simulink model "soft_continuum_model_2_sec"  (R2022a)
settings: Solver=VariableStepAuto  StartTime=0.0  StopTime=4  FixedStep=0.1  RelTol=1e-2
values from neighbouring files (symbols this model uses):
  D = diag([D_1,D_2,D_3,D_4,D_5,D_6])    [workspace_variables.m]
  E_1 = 8.25 * 10^4    (= 82500)    [workspace_variables.m]
  E_2 = 8.25 * 10^4    (= 82500)    [workspace_variables.m]
  g = [g_x,g_y,g_z]    [workspace_variables.m]
  Gs_1 = E_1 / ( 2 * ( 1 + ni) )    (= 27500)    [workspace_variables.m]
  Gs_2 = E_2 / ( 2 *( 1 + ni) )    (= 27500)    [workspace_variables.m]
  Ia_1 = diag([Iax_1,Iay_1,Iaz_1])    [workspace_variables.m]
  Ia_2 = diag([Iax_2,Iay_2,Iaz_2])    [workspace_variables.m]
  Im_1 = diag([Imx_1,Imy_1,Imz_1])    [workspace_variables.m]
  Im_2 = diag([Imx_2,Imy_2,Imz_2])    [workspace_variables.m]
  l_1 = 0.05    [workspace_variables.m]
  l_2 = 0.05    [workspace_variables.m]
  m_1 = 0.08    [workspace_variables.m]
  m_2 = 0.08    [workspace_variables.m]
  q_0 = [0.01 , 0 , 0 , 0.001, 0, 0.0]'    [workspace_variables.m]
  q_dot_0 = [0 , 0, 0, 0, 0, 0]'    [workspace_variables.m]
  t1_p = [0.025  , 0 , 0]    [workspace_variables.m]
  t2_p = [-0.025  , 0 , 0]    [workspace_variables.m]
  t3_p = [0  , 0.025 , 0]    [workspace_variables.m]
  t4_p = [0  , -0.025 , 0]    [workspace_variables.m]
  t5_p = [0.015  , 0 , 0]    [workspace_variables.m]
  twt = pi / 4    (= 0.785398163397)    [workspace_variables.m]
libraries: matrix_library x4, slpidlib x3, dspinverses x3
(part 2 of 2)

== matlab function soft_continuum_model_2_sec/robot model/Subsystem/MATLAB Function1 ==
  data: A input; y output
function y = fcn(A)
 y = cond(A)

== matlab function soft_continuum_model_2_sec/control/PD/Tendons1/Tendons/Subsystem/MATLAB Function1 ==
  data: q input; T_01 output; T_02 output; l_1 input; l_2 input
function [T_01,T_02] = fcn(q,l_1,l_2)
    k_1 = q(1);
    b_1 = q(2);
    t_1 = q(3);
    k_2 = q(4);
    b_2 = q(5);
    t_2 = q(6);
    T1 = T_1(b_1,k_1,l_1,t_1);
    T2 = T_2(b_2,k_2,l_2,t_2);

    T_01 = T1;
    T_02 = T1 * T2;

== matlab function soft_continuum_model_2_sec/Subsystem/Subsystem1/MATLAB Function ==
  data: m_1 input; J1_n output; J2_n output; G_n output; B_n output; C_n output; D_n output; m_2 input; Im_1 input; Im_2 input; l_1 input; l_2 input; Ia_1 input; Ia_2 input; D input; E_1 input; E_2 input; Gs_1 input; Gs_2 input; g input; q input; q_dot input
function [J1_n,J2_n,G_n,B_n,C_n,D_n] = DYNAMIC_MATRICES(m_1,m_2,Im_1,Im_2,l_1,l_2,Ia_1,Ia_2,D,E_1,E_2,Gs_1,Gs_2,g,q,q_dot)

k_1 = q(1);
b_1 = q(2);
t_1 = q(3);
k_2 = q(4);
b_2 = q(5);
t_2 = q(6);

k_dot_1 = q_dot(1);
b_dot_1 = q_dot(2);
t_dot_1 = q_dot(3);
k_dot_2 = q_dot(4);
b_dot_2 = q_dot(5);
t_dot_2 = q_dot(6);

Iax_1 = Ia_1(1,1);
Iay_1 = Ia_1(2,2);
Iaz_1 = Ia_1(3,3);

Iax_2 = Ia_2(1,1);
Iay_2 = Ia_2(2,2);
Iaz_2 = Ia_2(3,3);

Imx_1 = Im_1(1,1);
Imy_1 = Im_1(2,2);
Imz_1 = Im_1(3,3);

Imx_2 = Im_2(1,1);
Imy_2 = Im_2(2,2);
Imz_2 = Im_2(3,3);


g_x = g(1);
g_y = g(2);
g_z = g(3);

C_1_1 = C11(Imx_1,Imx_2,Imy_1,Imy_2,Imz_1,Imz_2,b_1,b_2,b_dot_1,b_dot_2,k_1,k_2,k_dot_1,k_dot_2,l_1,l_2,m_1,m_2,t_1,t_2,t_dot_1,t_dot_2);
C_1_2 = C12(Imx_1,Imx_2,Imy_1,Imy_2,Imz_1,Imz_2,b_1,b_2,b_dot_1,b_dot_2,k_1,k_2,k_dot_1,k_dot_2,l_1,l_2,m_1,m_2,t_1,t_2,t_dot_1,t_dot_2);
C_1_3 = C13(Imx_1,Imx_2,Imy_1,Imy_2,Imz_1,Imz_2,b_1,b_2,b_dot_1,b_dot_2,k_1,k_2,k_dot_1,k_dot_2,l_1,l_2,m_1,m_2,t_1,t_2,t_dot_1,t_dot_2);
C_1_4 = C14(Imx_2,Imy_2,Imz_2,b_1,b_2,b_dot_1,b_dot_2,k_1,k_2,k_dot_1,k_dot_2,l_1,l_2,m_2,t_1,t_2,t_dot_1,t_dot_2);
C_1_5 = C15(Imx_2,Imy_2,Imz_2,b_1,b_2,b_dot_1,b_dot_2,k_1,k_2,k_dot_1,k_dot_2,l_1,l_2,m_2,t_1,t_2,t_dot_1,t_dot_2);
C_1_6 = C16(Imx_2,Imy_2,Imz_2,b_1,b_2,b_dot_1,b_dot_2,k_1,k_2,k_dot_1,k_dot_2,l_1,l_2,m_2,t_1,t_2,t_dot_1,t_dot_2);

C_2_1 = C21(Imx_1,Imx_2,Imy_1,Imy_2,Imz_1,Imz_2,b_1,b_2,b_dot_1,b_dot_2,k_1,k_2,k_dot_1,k_dot_2,l_1,l_2,m_1,m_2,t_1,t_2,t_dot_1,t_dot_2);
C_2_2 = C21(Imx_1,Imx_2,Imy_1,Imy_2,Imz_1,Imz_2,b_1,b_2,b_dot_1,b_dot_2,k_1,k_2,k_dot_1,k_dot_2,l_1,l_2,m_1,m_2,t_1,t_2,t_dot_1,t_dot_2);
C_2_3 = C21(Imx_1,Imx_2,Imy_1,Imy_2,Imz_1,Imz_2,b_1,b_2,b_dot_1,b_dot_2,k_1,k_2,k_dot_1,k_dot_2,l_1,l_2,m_1,m_2,t_1,t_2,t_dot_1,t_dot_2);
C_2_4 = C26(Imx_2,Imy_2,Imz_2,b_1,b_2,b_dot_1,b_dot_2,k_1,k_2,k_dot_1,k_dot_2,l_1,l_2,m_2,t_1,t_2,t_dot_1,t_dot_2);
C_2_5 = C26(Imx_2,Imy_2,Imz_2,b_1,b_2,b_dot_1,b_dot_2,k_1,k_2,k_dot_1,k_dot_2,l_1,l_2,m_2,t_1,t_2,t_dot_1,t_dot_2);
C_2_6 = C26(Imx_2,Imy_2,Imz_2,b_1,b_2,b_dot_1,b_dot_2,k_1,k_2,k_dot_1,k_dot_2,l_1,l_2,m_2,t_1,t_2,t_dot_1,t_dot_2);

C_3_1 = C31(Imx_1,Imx_2,Imy_1,Imy_2,Imz_1,Imz_2,b_1,b_2,b_dot_1,b_dot_2,k_1,k_2,k_dot_1,k_dot_2,l_1,l_2,m_1,m_2,t_1,t_2,t_dot_1,t_dot_2);
C_3_2 = C32(Imx_1,Imx_2,Imy_1,Imy_2,Imz_1,Imz_2,b_1,b_2,b_dot_1,b_dot_2,k_1,k_2,k_dot_1,k_dot_2,l_1,l_2,m_1,m_2,t_1,t_2,t_dot_1,t_dot_2);
C_3_3 = C33(Imx_1,Imx_2,Imy_1,Imy_2,Imz_1,Imz_2,b_1,b_2,b_dot_1,b_dot_2,k_1,k_2,k_dot_1,k_dot_2,l_1,l_2,m_1,m_2,t_1,t_2,t_dot_1,t_dot_2);
C_3_4 =C34(Imx_2,Imy_2,Imz_2,b_1,b_2,b_dot_1,b_dot_2,k_1,k_2,k_dot_1,k_dot_2,l_1,l_2,m_2,t_1,t_2,t_dot_1,t_dot_2);
C_3_5 = C35(Imx_2,Imy_2,Imz_2,b_1,b_2,b_dot_1,b_dot_2,k_1,k_2,k_dot_1,k_dot_2,l_1,l_2,m_2,t_1,t_2,t_dot_1,t_dot_2);
C_3_6 =C36(Imx_2,Imy_2,Imz_2,b_1,b_2,b_dot_1,b_dot_2,k_1,k_2,k_dot_1,k_dot_2,l_1,l_2,m_2,t_1,t_2,t_dot_1,t_dot_2);

C_4_1 = C41(Imx_2,Imy_2,Imz_2,b_1,b_2,b_dot_1,b_dot_2,k_1,k_2,k_dot_1,k_dot_2,l_1,l_2,m_2,t_1,t_2,t_dot_1,t_dot_2);
C_4_2 = C42(Imx_2,Imy_2,Imz_2,b_1,b_2,b_dot_1,b_dot_2,k_1,k_2,k_dot_1,k_dot_2,l_1,l_2,m_2,t_1,t_2,t_dot_1,t_dot_2);
C_4_3 =C43(Imx_2,Imy_2,Imz_2,b_1,b_2,b_dot_1,b_dot_2,k_1,k_2,k_dot_1,k_dot_2,l_1,l_2,m_2,t_1,t_2,t_dot_1,t_dot_2);
C_4_4 =C44(Imx_2,Imy_2,Imz_2,b_1,b_2,b_dot_1,b_dot_2,k_1,k_2,k_dot_1,k_dot_2,l_1,l_2,m_2,t_1,t_2,t_dot_1,t_dot_2);
C_4_5 =C45(Imx_2,Imy_2,Imz_2,b_1,b_2,b_dot_1,b_dot_2,k_1,k_2,k_dot_1,k_dot_2,l_1,l_2,m_2,t_1,t_2,t_dot_1,t_dot_2);
C_4_6 =C46(Imx_2,Imy_2,Imz_2,b_1,b_2,b_dot_1,b_dot_2,k_1,k_2,k_dot_1,k_dot_2,l_1,l_2,m_2,t_1,t_2,t_dot_1,t_dot_2);

C_5_1 =C51(Imx_2,Imy_2,Imz_2,b_1,b_2,b_dot_1,b_dot_2,k_1,k_2,k_dot_1,k_dot_2,l_1,l_2,m_2,t_1,t_2,t_dot_1,t_dot_2);
C_5_2 = C52(Imx_2,Imy_2,Imz_2,b_1,b_2,b_dot_1,b_dot_2,k_1,k_2,k_dot_1,k_dot_2,l_1,l_2,m_2,t_1,t_2,t_dot_1,t_dot_2);
C_5_3 =C53(Imx_2,Imy_2,Imz_2,b_1,b_2,b_dot_1,b_dot_2,k_1,k_2,k_dot_1,k_dot_2,l_1,l_2,m_2,t_1,t_2,t_dot_1,t_dot_2);
C_5_4 =C54(Imx_2,Imy_2,Imz_2,b_1,b_2,b_dot_1,b_dot_2,k_1,k_2,k_dot_1,k_dot_2,l_1,l_2,m_2,t_1,t_2,t_dot_1,t_dot_2);
C_5_5 =C55(Imx_2,Imy_2,Imz_2,b_1,b_2,b_dot_1,b_dot_2,k_1,k_2,k_dot_1,k_dot_2,l_1,l_2,m_2,t_1,t_2,t_dot_1,t_dot_2);
C_5_6 =C56(Imx_2,Imy_2,Imz_2,b_1,b_2,b_dot_1,b_dot_2,k_1,k_2,k_dot_1,k_dot_2,l_1,l_2,m_2,t_1,t_2,t_dot_1,t_dot_2);

C_6_1 =C61(Imx_2,Imy_2,Imz_2,b_1,b_2,b_dot_1,b_dot_2,k_1,k_2,k_dot_1,k_dot_2,l_1,l_2,m_2,t_1,t_2,t_dot_1,t_dot_2);
C_6_2 = C62(Imx_2,Imy_2,Imz_2,b_1,b_2,b_dot_1,b_dot_2,k_1,k_2,k_dot_1,k_dot_2,l_1,l_2,m_2,t_1,t_2,t_dot_1,t_dot_2);
C_6_3 =C63(Imx_2,Imy_2,Imz_2,b_1,b_2,b_dot_1,b_dot_2,k_1,k_2,k_dot_1,k_dot_2,l_1,l_2,m_2,t_1,t_2,t_dot_1,t_dot_2);
C_6_4 =C64(Imx_2,Imy_2,Imz_2,b_1,b_2,b_dot_1,b_dot_2,k_1,k_2,k_dot_1,k_dot_2,l_1,l_2,m_2,t_1,t_2,t_dot_1,t_dot_2);
C_6_5 =C65(Imx_2,Imy_2,Imz_2,b_1,b_2,b_dot_1,b_dot_2,k_1,k_2,k_dot_1,k_dot_2,l_1,l_2,m_2,t_1,t_2,t_dot_1,t_dot_2);
C_6_6 =C66(Imx_2,Imy_2,Imz_2,b_1,b_2,b_dot_1,b_dot_2,k_1,k_2,k_dot_1,k_dot_2,l_1,l_2,m_2,t_1,t_2,t_dot_1,t_dot_2);

C_n = [ C_1_1,C_1_2,C_1_3,C_1_4,C_1_5,C_1_6;
        C_2_1,C_2_2,C_2_3,C_2_4,C_2_5,C_2_6;
        C_3_1,C_3_2,C_3_3,C_3_4,C_3_5,C_3_6;
        C_4_1,C_4_2,C_4_3,C_4_4,C_4_5,C_4_6;
        C_5_1,C_5_2,C_5_3,C_5_4,C_5_5,C_5_6;
        C_6_1,C_6_2,C_6_3,C_6_4,C_6_5,C_6_6;
      ];
 J1_n= J_1(b_1,k_1,l_1,t_1);
 J2_n= J_2(b_1,b_2,k_1,k_2,l_1,l_2,t_1,t_2);
 B_n=B(Imx_1,Imx_2,Imy_1,Imy_2,Imz_1,Imz_2,b_1,b_2,k_1,k_2,l_1,l_2,m_1,m_2,t_1,t_2);
 G_n =G(E_1,E_2,Gs_1,Gs_2,Iax_1,Iax_2,Iay_1,Iay_2,Iaz_1,Iaz_2,b_1,b_2,g_x,g_y,g_z,k_1,k_2,l_1,l_2,m_1,m_2,t_1,t_2);
D_n = D;

== matlab function soft_continuum_model_2_sec/robot model/Subsystem2/matrices/MATLAB Function ==
  data: m_1 input; J1_n output; J2_n output; G_n output; B_n output; C_n output; D_n output; m_2 input; Im_1 input; Im_2 input; l_1 input; l_2 input; Ia_1 input; Ia_2 input; D input; E_1 input; E_2 input; Gs_1 input; Gs_2 input; g input; q input; q_dot input
function [J1_n,J2_n,G_n,B_n,C_n,D_n] = dynamics_matrices(m_1,m_2,Im_1,Im_2,l_1,l_2,Ia_1,Ia_2,D,E_1,E_2,Gs_1,Gs_2,g,q,q_dot)

k_1 = q(1);
b_1 = q(2);
t_1 = q(3);
k_2 = q(4);
b_2 = q(5);
t_2 = q(6);

k_dot_1 = q_dot(1);
b_dot_1 = q_dot(2);
t_dot_1 = q_dot(3);
k_dot_2 = q_dot(4);
b_dot_2 = q_dot(5);
t_dot_2 = q_dot(6);

Iax_1 = Ia_1(1,1);
Iay_1 = Ia_1(2,2);
Iaz_1 = Ia_1(3,3);

Iax_2 = Ia_2(1,1);
Iay_2 = Ia_2(2,2);
Iaz_2 = Ia_2(3,3);

Imx_1 = Im_1(1,1);
Imy_1 = Im_1(2,2);
Imz_1 = Im_1(3,3);

Imx_2 = Im_2(1,1);
Imy_2 = Im_2(2,2);
Imz_2 = Im_2(3,3);

A = 0;
A_2 = 0;

g_x = g(1);
g_y = g(2);
g_z = g(3);

C_1_1 = C11(k_1,b_1,t_1,k_2,b_2,t_2,k_dot_1,b_dot_1,t_dot_1,k_dot_2,b_dot_2,t_dot_2,l_1,l_2,A,A_2,Iax_2,Iay_2,Iaz_2,Iax_1,Iay_1,Iaz_1,Imx_1,Imy_1,Imz_1,Imx_2,Imy_2,Imz_2,m_1,m_2,g_x,g_y,g_z,Gs_1,E_1,Gs_2,E_2);
C_1_2 = C12(k_1,b_1,t_1,k_2,b_2,t_2,k_dot_1,b_dot_1,t_dot_1,k_dot_2,b_dot_2,t_dot_2,l_1,l_2,A,A_2,Iax_2,Iay_2,Iaz_2,Iax_1,Iay_1,Iaz_1,Imx_1,Imy_1,Imz_1,Imx_2,Imy_2,Imz_2,m_1,m_2,g_x,g_y,g_z,Gs_1,E_1,Gs_2,E_2);
C_1_3 = C13(k_1,b_1,t_1,k_2,b_2,t_2,k_dot_1,b_dot_1,t_dot_1,k_dot_2,b_dot_2,t_dot_2,l_1,l_2,A,A_2,Iax_2,Iay_2,Iaz_2,Iax_1,Iay_1,Iaz_1,Imx_1,Imy_1,Imz_1,Imx_2,Imy_2,Imz_2,m_1,m_2,g_x,g_y,g_z,Gs_1,E_1,Gs_2,E_2);
C_1_4 = C14(k_1,b_1,t_1,k_2,b_2,t_2,k_dot_1,b_dot_1,t_dot_1,k_dot_2,b_dot_2,t_dot_2,l_1,l_2,A,A_2,Iax_2,Iay_2,Iaz_2,Iax_1,Iay_1,Iaz_1,Imx_1,Imy_1,Imz_1,Imx_2,Imy_2,Imz_2,m_1,m_2,g_x,g_y,g_z,Gs_1,E_1,Gs_2,E_2);
C_1_5 = C15(k_1,b_1,t_1,k_2,b_2,t_2,k_dot_1,b_dot_1,t_dot_1,k_dot_2,b_dot_2,t_dot_2,l_1,l_2,A,A_2,Iax_2,Iay_2,Iaz_2,Iax_1,Iay_1,Iaz_1,Imx_1,Imy_1,Imz_1,Imx_2,Imy_2,Imz_2,m_1,m_2,g_x,g_y,g_z,Gs_1,E_1,Gs_2,E_2);
C_1_6 = C16(k_1,b_1,t_1,k_2,b_2,t_2,k_dot_1,b_dot_1,t_dot_1,k_dot_2,b_dot_2,t_dot_2,l_1,l_2,A,A_2,Iax_2,Iay_2,Iaz_2,Iax_1,Iay_1,Iaz_1,Imx_1,Imy_1,Imz_1,Imx_2,Imy_2,Imz_2,m_1,m_2,g_x,g_y,g_z,Gs_1,E_1,Gs_2,E_2);

C_2_1 = C21(k_1,b_1,t_1,k_2,b_2,t_2,k_dot_1,b_dot_1,t_dot_1,k_dot_2,b_dot_2,t_dot_2,l_1,l_2,A,A_2,Iax_2,Iay_2,Iaz_2,Iax_1,Iay_1,Iaz_1,Imx_1,Imy_1,Imz_1,Imx_2,Imy_2,Imz_2,m_1,m_2,g_x,g_y,g_z,Gs_1,E_1,Gs_2,E_2);
C_2_2 = C21(k_1,b_1,t_1,k_2,b_2,t_2,k_dot_1,b_dot_1,t_dot_1,k_dot_2,b_dot_2,t_dot_2,l_1,l_2,A,A_2,Iax_2,Iay_2,Iaz_2,Iax_1,Iay_1,Iaz_1,Imx_1,Imy_1,Imz_1,Imx_2,Imy_2,Imz_2,m_1,m_2,g_x,g_y,g_z,Gs_1,E_1,Gs_2,E_2);
C_2_3 = C21(k_1,b_1,t_1,k_2,b_2,t_2,k_dot_1,b_dot_1,t_dot_1,k_dot_2,b_dot_2,t_dot_2,l_1,l_2,A,A_2,Iax_2,Iay_2,Iaz_2,Iax_1,Iay_1,Iaz_1,Imx_1,Imy_1,Imz_1,Imx_2,Imy_2,Imz_2,m_1,m_2,g_x,g_y,g_z,Gs_1,E_1,Gs_2,E_2);
C_2_4 = C26(k_1,b_1,t_1,k_2,b_2,t_2,k_dot_1,b_dot_1,t_dot_1,k_dot_2,b_dot_2,t_dot_2,l_1,l_2,A,A_2,Iax_2,Iay_2,Iaz_2,Iax_1,Iay_1,Iaz_1,Imx_1,Imy_1,Imz_1,Imx_2,Imy_2,Imz_2,m_1,m_2,g_x,g_y,g_z,Gs_1,E_1,Gs_2,E_2);
C_2_5 = C26(k_1,b_1,t_1,k_2,b_2,t_2,k_dot_1,b_dot_1,t_dot_1,k_dot_2,b_dot_2,t_dot_2,l_1,l_2,A,A_2,Iax_2,Iay_2,Iaz_2,Iax_1,Iay_1,Iaz_1,Imx_1,Imy_1,Imz_1,Imx_2,Imy_2,Imz_2,m_1,m_2,g_x,g_y,g_z,Gs_1,E_1,Gs_2,E_2);
C_2_6 = C26(k_1,b_1,t_1,k_2,b_2,t_2,k_dot_1,b_dot_1,t_dot_1,k_dot_2,b_dot_2,t_dot_2,l_1,l_2,A,A_2,Iax_2,Iay_2,Iaz_2,Iax_1,Iay_1,Iaz_1,Imx_1,Imy_1,Imz_1,Imx_2,Imy_2,Imz_2,m_1,m_2,g_x,g_y,g_z,Gs_1,E_1,Gs_2,E_2);

C_3_1 = C31(k_1,b_1,t_1,k_2,b_2,t_2,k_dot_1,b_dot_1,t_dot_1,k_dot_2,b_dot_2,t_dot_2,l_1,l_2,A,A_2,Iax_2,Iay_2,Iaz_2,Iax_1,Iay_1,Iaz_1,Imx_1,Imy_1,Imz_1,Imx_2,Imy_2,Imz_2,m_1,m_2,g_x,g_y,g_z,Gs_1,E_1,Gs_2,E_2);
C_3_2 = C32(k_1,b_1,t_1,k_2,b_2,t_2,k_dot_1,b_dot_1,t_dot_1,k_dot_2,b_dot_2,t_dot_2,l_1,l_2,A,A_2,Iax_2,Iay_2,Iaz_2,Iax_1,Iay_1,Iaz_1,Imx_1,Imy_1,Imz_1,Imx_2,Imy_2,Imz_2,m_1,m_2,g_x,g_y,g_z,Gs_1,E_1,Gs_2,E_2);
C_3_3 = C33(k_1,b_1,t_1,k_2,b_2,t_2,k_dot_1,b_dot_1,t_dot_1,k_dot_2,b_dot_2,t_dot_2,l_1,l_2,A,A_2,Iax_2,Iay_2,Iaz_2,Iax_1,Iay_1,Iaz_1,Imx_1,Imy_1,Imz_1,Imx_2,Imy_2,Imz_2,m_1,m_2,g_x,g_y,g_z,Gs_1,E_1,Gs_2,E_2);
C_3_4 =C34(k_1,b_1,t_1,k_2,b_2,t_2,k_dot_1,b_dot_1,t_dot_1,k_dot_2,b_dot_2,t_dot_2,l_1,l_2,A,A_2,Iax_2,Iay_2,Iaz_2,Iax_1,Iay_1,Iaz_1,Imx_1,Imy_1,Imz_1,Imx_2,Imy_2,Imz_2,m_1,m_2,g_x,g_y,g_z,Gs_1,E_1,Gs_2,E_2);
C_3_5 = C35(k_1,b_1,t_1,k_2,b_2,t_2,k_dot_1,b_dot_1,t_dot_1,k_dot_2,b_dot_2,t_dot_2,l_1,l_2,A,A_2,Iax_2,Iay_2,Iaz_2,Iax_1,Iay_1,Iaz_1,Imx_1,Imy_1,Imz_1,Imx_2,Imy_2,Imz_2,m_1,m_2,g_x,g_y,g_z,Gs_1,E_1,Gs_2,E_2);
C_3_6 =C36(k_1,b_1,t_1,k_2,b_2,t_2,k_dot_1,b_dot_1,t_dot_1,k_dot_2,b_dot_2,t_dot_2,l_1,l_2,A,A_2,Iax_2,Iay_2,Iaz_2,Iax_1,Iay_1,Iaz_1,Imx_1,Imy_1,Imz_1,Imx_2,Imy_2,Imz_2,m_1,m_2,g_x,g_y,g_z,Gs_1,E_1,Gs_2,E_2);

C_4_1 = C41(k_1,b_1,t_1,k_2,b_2,t_2,k_dot_1,b_dot_1,t_dot_1,k_dot_2,b_dot_2,t_dot_2,l_1,l_2,A,A_2,Iax_2,Iay_2,Iaz_2,Iax_1,Iay_1,Iaz_1,Imx_1,Imy_1,Imz_1,Imx_2,Imy_2,Imz_2,m_1,m_2,g_x,g_y,g_z,Gs_1,E_1,Gs_2,E_2);
C_4_2 = C42(k_1,b_1,t_1,k_2,b_2,t_2,k_dot_1,b_dot_1,t_dot_1,k_dot_2,b_dot_2,t_dot_2,l_1,l_2,A,A_2,Iax_2,Iay_2,Iaz_2,Iax_1,Iay_1,Iaz_1,Imx_1,Imy_1,Imz_1,Imx_2,Imy_2,Imz_2,m_1,m_2,g_x,g_y,g_z,Gs_1,E_1,Gs_2,E_2);
C_4_3 =C43(k_1,b_1,t_1,k_2,b_2,t_2,k_dot_1,b_dot_1,t_dot_1,k_dot_2,b_dot_2,t_dot_2,l_1,l_2,A,A_2,Iax_2,Iay_2,Iaz_2,Iax_1,Iay_1,Iaz_1,Imx_1,Imy_1,Imz_1,Imx_2,Imy_2,Imz_2,m_1,m_2,g_x,g_y,g_z,Gs_1,E_1,Gs_2,E_2);
C_4_4 =C44(k_1,b_1,t_1,k_2,b_2,t_2,k_dot_1,b_dot_1,t_dot_1,k_dot_2,b_dot_2,t_dot_2,l_1,l_2,A,A_2,Iax_2,Iay_2,Iaz_2,Iax_1,Iay_1,Iaz_1,Imx_1,Imy_1,Imz_1,Imx_2,Imy_2,Imz_2,m_1,m_2,g_x,g_y,g_z,Gs_1,E_1,Gs_2,E_2);
C_4_5 =C45(k_1,b_1,t_1,k_2,b_2,t_2,k_dot_1,b_dot_1,t_dot_1,k_dot_2,b_dot_2,t_dot_2,l_1,l_2,A,A_2,Iax_2,Iay_2,Iaz_2,Iax_1,Iay_1,Iaz_1,Imx_1,Imy_1,Imz_1,Imx_2,Imy_2,Imz_2,m_1,m_2,g_x,g_y,g_z,Gs_1,E_1,Gs_2,E_2);
C_4_6 =C46(k_1,b_1,t_1,k_2,b_2,t_2,k_dot_1,b_dot_1,t_dot_1,k_dot_2,b_dot_2,t_dot_2,l_1,l_2,A,A_2,Iax_2,Iay_2,Iaz_2,Iax_1,Iay_1,Iaz_1,Imx_1,Imy_1,Imz_1,Imx_2,Imy_2,Imz_2,m_1,m_2,g_x,g_y,g_z,Gs_1,E_1,Gs_2,E_2);

C_5_1 =C51(k_1,b_1,t_1,k_2,b_2,t_2,k_dot_1,b_dot_1,t_dot_1,k_dot_2,b_dot_2,t_dot_2,l_1,l_2,A,A_2,Iax_2,Iay_2,Iaz_2,Iax_1,Iay_1,Iaz_1,Imx_1,Imy_1,Imz_1,Imx_2,Imy_2,Imz_2,m_1,m_2,g_x,g_y,g_z,Gs_1,E_1,Gs_2,E_2);
C_5_2 = C52(k_1,b_1,t_1,k_2,b_2,t_2,k_dot_1,b_dot_1,t_dot_1,k_dot_2,b_dot_2,t_dot_2,l_1,l_2,A,A_2,Iax_2,Iay_2,Iaz_2,Iax_1,Iay_1,Iaz_1,Imx_1,Imy_1,Imz_1,Imx_2,Imy_2,Imz_2,m_1,m_2,g_x,g_y,g_z,Gs_1,E_1,Gs_2,E_2);
C_5_3 =C53(k_1,b_1,t_1,k_2,b_2,t_2,k_dot_1,b_dot_1,t_dot_1,k_dot_2,b_dot_2,t_dot_2,l_1,l_2,A,A_2,Iax_2,Iay_2,Iaz_2,Iax_1,Iay_1,Iaz_1,Imx_1,Imy_1,Imz_1,Imx_2,Imy_2,Imz_2,m_1,m_2,g_x,g_y,g_z,Gs_1,E_1,Gs_2,E_2);
C_5_4 =C54(k_1,b_1,t_1,k_2,b_2,t_2,k_dot_1,b_dot_1,t_dot_1,k_dot_2,b_dot_2,t_dot_2,l_1,l_2,A,A_2,Iax_2,Iay_2,Iaz_2,Iax_1,Iay_1,Iaz_1,Imx_1,Imy_1,Imz_1,Imx_2,Imy_2,Imz_2,m_1,m_2,g_x,g_y,g_z,Gs_1,E_1,Gs_2,E_2);
C_5_5 =C55(k_1,b_1,t_1,k_2,b_2,t_2,k_dot_1,b_dot_1,t_dot_1,k_dot_2,b_dot_2,t_dot_2,l_1,l_2,A,A_2,Iax_2,Iay_2,Iaz_2,Iax_1,Iay_1,Iaz_1,Imx_1,Imy_1,Imz_1,Imx_2,Imy_2,Imz_2,m_1,m_2,g_x,g_y,g_z,Gs_1,E_1,Gs_2,E_2);
C_5_6 =C56(k_1,b_1,t_1,k_2,b_2,t_2,k_dot_1,b_dot_1,t_dot_1,k_dot_2,b_dot_2,t_dot_2,l_1,l_2,A,A_2,Iax_2,Iay_2,Iaz_2,Iax_1,Iay_1,Iaz_1,Imx_1,Imy_1,Imz_1,Imx_2,Imy_2,Imz_2,m_1,m_2,g_x,g_y,g_z,Gs_1,E_1,Gs_2,E_2);

C_6_1 =C61(k_1,b_1,t_1,k_2,b_2,t_2,k_dot_1,b_dot_1,t_dot_1,k_dot_2,b_dot_2,t_dot_2,l_1,l_2,A,A_2,Iax_2,Iay_2,Iaz_2,Iax_1,Iay_1,Iaz_1,Imx_1,Imy_1,Imz_1,Imx_2,Imy_2,Imz_2,m_1,m_2,g_x,g_y,g_z,Gs_1,E_1,Gs_2,E_2);
C_6_2 = C62(k_1,b_1,t_1,k_2,b_2,t_2,k_dot_1,b_dot_1,t_dot_1,k_dot_2,b_dot_2,t_dot_2,l_1,l_2,A,A_2,Iax_2,Iay_2,Iaz_2,Iax_1,Iay_1,Iaz_1,Imx_1,Imy_1,Imz_1,Imx_2,Imy_2,Imz_2,m_1,m_2,g_x,g_y,g_z,Gs_1,E_1,Gs_2,E_2);
C_6_3 =C63(k_1,b_1,t_1,k_2,b_2,t_2,k_dot_1,b_dot_1,t_dot_1,k_dot_2,b_dot_2,t_dot_2,l_1,l_2,A,A_2,Iax_2,Iay_2,Iaz_2,Iax_1,Iay_1,Iaz_1,Imx_1,Imy_1,Imz_1,Imx_2,Imy_2,Imz_2,m_1,m_2,g_x,g_y,g_z,Gs_1,E_1,Gs_2,E_2);
C_6_4 =C64(k_1,b_1,t_1,k_2,b_2,t_2,k_dot_1,b_dot_1,t_dot_1,k_dot_2,b_dot_2,t_dot_2,l_1,l_2,A,A_2,Iax_2,Iay_2,Iaz_2,Iax_1,Iay_1,Iaz_1,Imx_1,Imy_1,Imz_1,Imx_2,Imy_2,Imz_2,m_1,m_2,g_x,g_y,g_z,Gs_1,E_1,Gs_2,E_2);
C_6_5 =C65(k_1,b_1,t_1,k_2,b_2,t_2,k_dot_1,b_dot_1,t_dot_1,k_dot_2,b_dot_2,t_dot_2,l_1,l_2,A,A_2,Iax_2,Iay_2,Iaz_2,Iax_1,Iay_1,Iaz_1,Imx_1,Imy_1,Imz_1,Imx_2,Imy_2,Imz_2,m_1,m_2,g_x,g_y,g_z,Gs_1,E_1,Gs_2,E_2);
C_6_6 =C66(k_1,b_1,t_1,k_2,b_2,t_2,k_dot_1,b_dot_1,t_dot_1,k_dot_2,b_dot_2,t_dot_2,l_1,l_2,A,A_2,Iax_2,Iay_2,Iaz_2,Iax_1,Iay_1,Iaz_1,Imx_1,Imy_1,Imz_1,Imx_2,Imy_2,Imz_2,m_1,m_2,g_x,g_y,g_z,Gs_1,E_1,Gs_2,E_2);

C_n = [ C_1_1,C_1_2,C_1_3,C_1_4,C_1_5,C_1_6;
        C_2_1,C_2_2,C_2_3,C_2_4,C_2_5,C_2_6;
        C_3_1,C_3_2,C_3_3,C_3_4,C_3_5,C_3_6;
        C_4_1,C_4_2,C_4_3,C_4_4,C_4_5,C_4_6;
        C_5_1,C_5_2,C_5_3,C_5_4,C_5_5,C_5_6;
        C_6_1,C_6_2,C_6_3,C_6_4,C_6_5,C_6_6;
      ];
 J1_n= J_1(b_1,k_1,l_1,t_1);
 J2_n= J_2(b_1,b_2,k_1,k_2,l_1,l_2,t_1,t_2);
 B_n=B(k_1,b_1,t_1,k_2,b_2,t_2,k_dot_1,b_dot_1,t_dot_1,k_dot_2,b_dot_2,t_dot_2,l_1,l_2,A,A_2,Iax_2,Iay_2,Iaz_2,Iax_1,Iay_1,Iaz_1,Imx_1,Imy_1,Imz_1,Imx_2,Imy_2,Imz_2,m_1,m_2,g_x,g_y,g_z,Gs_1,E_1,Gs_2,E_2);
 G_n =G(k_1,b_1,t_1,k_2,b_2,t_2,k_dot_1,b_dot_1,t_dot_1,k_dot_2,b_dot_2,t_dot_2,l_1,l_2,A,A_2,Iax_2,Iay_2,Iaz_2,Iax_1,Iay_1,Iaz_1,Imx_1,Imy_1,Imz_1,Imx_2,Imy_2,Imz_2,m_1,m_2,g_x,g_y,g_z,Gs_1,E_1,Gs_2,E_2);
D_n = D;

== matlab function soft_continuum_model_2_sec/Subsystem/MATLAB Function ==
  data: u input; tensions output
function tensions = fcn(u)
    control_k_1 = u(1);
    control_b_1 = u(2);
    control_t_1 = u(3);
    control_k_2 = u(4);
    control_b_2 = u(5);
    control_t_2 = u(6);

    if control_k_2>= 0
        T_1 = control_k_2;
        T_2 = 0;
    else
        T_2 = control_k_2;
        T_1 = 0;
    end
    if control_b_2 >= 0
        T_3 = control_b_2;
        T_4 = 0;
    else
        T_4 = control_b_2;
        T_3 = 0;
    end
    if control_t_2>0
        T_5 = control_t_2;
    else 
        T_5 = 0;
    end
    tensions = [T_1 T_2 T_3 ,T_4 , T_5];

== matlab function soft_continuum_model_2_sec/Subsystem1/MATLAB Function1 ==
  data: q input; x output; l_1 input; l_2 input; y output; z output; roll output; pitch output; yaw output
function [x , y , z , roll , pitch ,yaw ] = fcn(q,l_1,l_2)
    k_1 = q(1);
    b_1 = q(2);
    t_1 = q(3);
    k_2 = q(4);
    b_2 = q(5);
    t_2 = q(6);
    T1 = T_1(b_1,k_1,l_1,t_1);
    T2 = T_2(b_2,k_2,l_2,t_2);

    T_01 = T1;
    tw = T1 * T2;

    x = tw(1,4) ;
    y = tw(2,4) ;
    z = tw(3,4) ;
    roll = tw(3,2) ;
    pitch = tw(1,3) ;
    yaw = tw(2,1) ;
